simulink model "helicopter_robust_controller"  (R2023b)
settings: Solver=VariableStepAuto  StartTime=0.0  StopTime=20  MaxStep=0.01  RelTol=1e-5
libraries: cstblocks x3
settings Model: Creator=torb  LastModifiedBy=torb

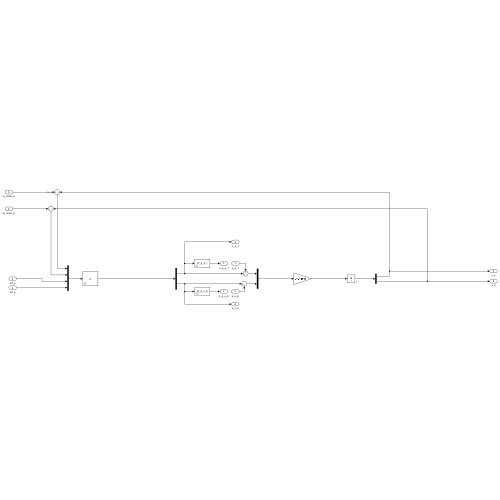
[thumbnail: Simulink's stored preview of the top-level diagram]
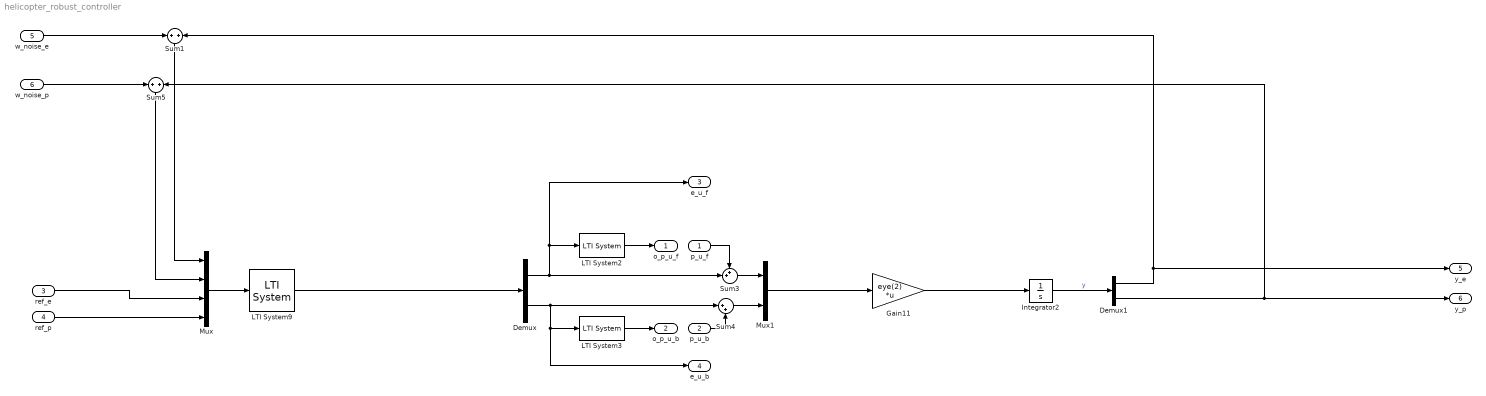
== system helicopter_robust_controller ==
  p_u_f : Inport
  p_u_b : Inport  Port=2
  ref_e : Inport  Port=3
  ref_p : Inport  Port=4
  w_noise_e : Inport  Port=5
  w_noise_p : Inport  Port=6
  Demux : Demux  Outputs=2
  Demux1 : Demux  Outputs=2
  Gain11 : Gain  Gain=eye(2)  Multiplication=Matrix(K*u)
  Integrator2 : Integrator
  LTI System2 : cstblocks/LTI System  sys=W_p_u_f  IC=[]  PadeOrder=0
  LTI System3 : cstblocks/LTI System  sys=W_p_u_b  IC=[]  PadeOrder=0
  LTI System9 : cstblocks/LTI System  sys=K  IC=[]  PadeOrder=0
  Mux : Mux
  Mux1 : Mux  Inputs=2
  Sum1 : Sum  Inputs=+|+
  Sum3 : Sum  Inputs=++|
  Sum4 : Sum  Inputs=|++
  Sum5 : Sum  Inputs=+|+
  o_p_u_f : Outport
  o_p_u_b : Outport  Port=2
  e_u_f : Outport  Port=3
  e_u_b : Outport  Port=4
  y_e : Outport  Port=5
  y_p : Outport  Port=6
  wires:
  Sum4/1 -> Mux1/2
  Demux/1 -> e_u_f/1, LTI System2/1, Sum3/2
  LTI System2/1 -> o_p_u_f/1
  ref_p/1 -> Mux/4
  p_u_b/1 -> Sum4/2
  LTI System3/1 -> o_p_u_b/1
  Demux1/2 -> y_p/1, Sum5/2
  Demux/2 -> Sum4/1, e_u_b/1, LTI System3/1
  p_u_f/1 -> Sum3/1
  Sum3/1 -> Mux1/1
  Integrator2/1 -> Demux1/1  "y"
  ref_e/1 -> Mux/3
  Demux1/1 -> y_e/1, Sum1/2
  Mux1/1 -> Gain11/1
  Gain11/1 -> Integrator2/1
  LTI System9/1 -> Demux/1
  Mux/1 -> LTI System9/1
  w_noise_e/1 -> Sum1/1
  Sum1/1 -> Mux/1
  w_noise_p/1 -> Sum5/1
  Sum5/1 -> Mux/2
